simulink model "mathematical_motor_model_2018"  (R2018a)
settings: Solver=VariableStepAuto  StartTime=0.0  StopTime=10.0  RelTol=1e-3
values from neighbouring files (symbols this model uses):
  b_m = 0.1    [motor_parameter.m]
  J = 0.01    [motor_parameter.m]
  Ke = 0.01    [motor_parameter.m]
  Km = 0.01    [motor_parameter.m]
  L = 0.5    [motor_parameter.m]
  R = 1    [motor_parameter.m]
settings Model: Creator=root  LastModifiedBy=root

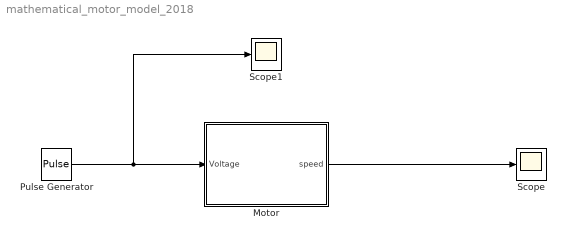
== system mathematical_motor_model_2018 ==
  Motor : Subsystem
  Pulse Generator : DiscretePulseGenerator  PulseType=Time based  Amplitude=1000  Period=10  PulseWidth=0.01
  Scope : Scope
  Scope1 : Scope
  wires:
  Pulse Generator/1 -> Scope1/1, Motor/1(Voltage)
  Motor/1(speed) -> Scope/1

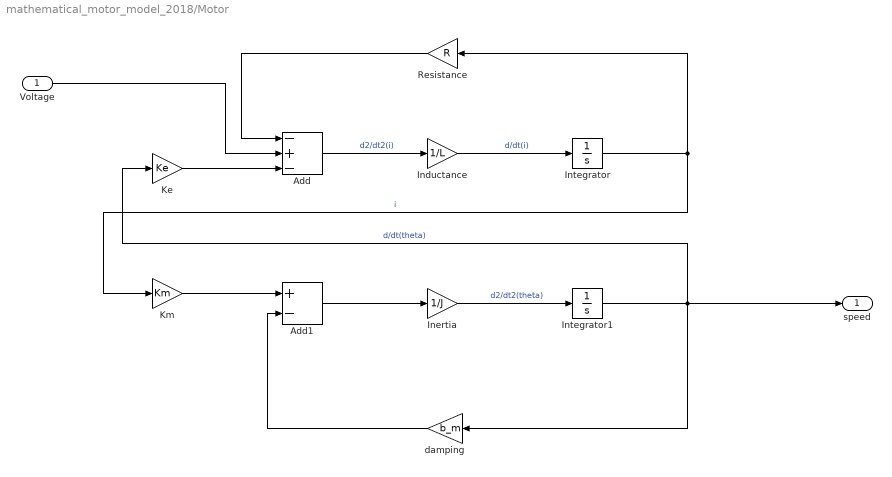
== system mathematical_motor_model_2018/Motor ==
  Voltage : Inport
  Add : Sum  Inputs=-+-
  Add1 : Sum  Inputs=+-
  Inductance : Gain  Gain=1/L
  Inertia : Gain  Gain=1/J
  Integrator : Integrator
  Integrator1 : Integrator
  Ke : Gain  Gain=Ke
  Km : Gain  Gain=Km
  Resistance : Gain  Gain=R
  damping : Gain  Gain=b_m
  speed : Outport
  wires:
  Voltage/1 -> Add/2
  Km/1 -> Add1/1
  Add/1 -> Inductance/1  "d2/dt2(i)"
  Inertia/1 -> Integrator1/1  "d2/dt2(theta)"
  damping/1 -> Add1/2
  Integrator1/1 -> speed/1, Ke/1, damping/1  "d/dt(theta)"
  Add1/1 -> Inertia/1
  Inductance/1 -> Integrator/1  "d/dt(i)"
  Resistance/1 -> Add/1
  Ke/1 -> Add/3
  Integrator/1 -> Resistance/1, Km/1  "i"
